simulink model "x3_2_F1_step_response"  (R2021b)
settings: Solver=VariableStepAuto  StartTime=0.0  StopTime=200  RelTol=1e-3
libraries: simulink x1
settings Model: Creator=Edwar  LastModifiedBy=Edwar

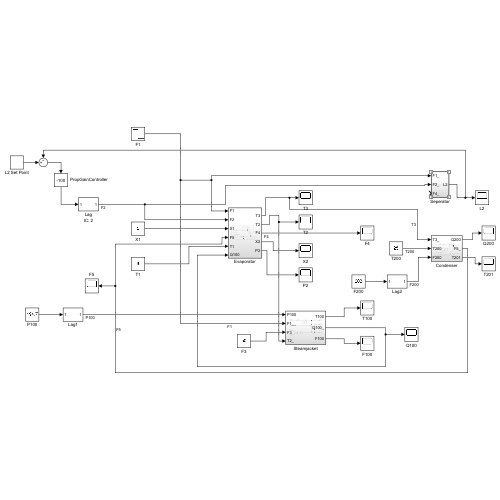
[thumbnail: Simulink's stored preview of the top-level diagram]
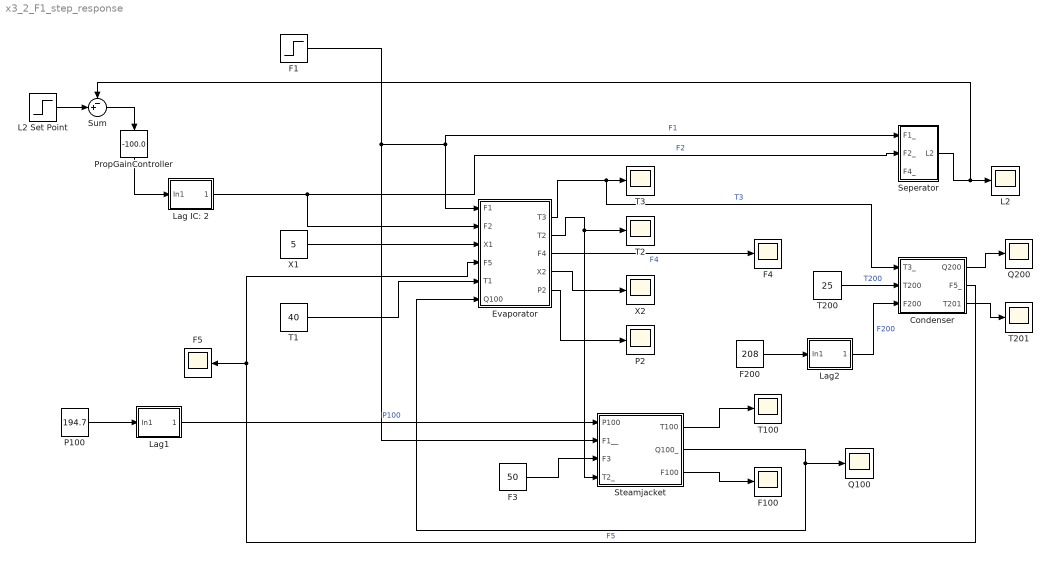
== system x3_2_F1_step_response ==
  Condenser : Subsystem
  Evaporator : Subsystem
  F1 : Step  Time=30  Before=10  After=9  SampleTime=0
  F100 : Scope
  F200 : Constant  Value=208
  F3 : Constant  Value=50
  F4 : Scope
  F5 : Scope
  L2 : Scope
  L2 Set Point : Step  Time=50  Before=1  SampleTime=0
  Lag IC: 2 : Subsystem
  Lag1 : Subsystem
  Lag2 : Subsystem
  P100 : Constant  Value=194.7
  P2 : Scope
  PropGainController : simulink/Math Operations/Slider Gain  gain=-100.0  low=-100  high=0
  Q100 : Scope
  Q200 : Scope
  Seperator : Subsystem
  Steamjacket : Subsystem
  Sum : Sum  Inputs=-+|
  T1 : Constant  Value=40
  T{2..3,100,201} (4 alike) : Scope
  T200 : Constant  Value=25
  X1 : Constant  Value=5
  X2 : Scope
  wires:
  Evaporator/2(T2) -> T2/1, Steamjacket/4(T2_)
  Steamjacket/3(F100) -> F100/1
  X1/1 -> Evaporator/3(X1)
  Evaporator/4(X2) -> X2/1
  F3/1 -> Steamjacket/3(F3)
  Steamjacket/2(Q100_) -> Q100/1, Evaporator/6(Q100)
  T1/1 -> Evaporator/5(T1)
  Condenser/1(Q200) -> Q200/1
  Evaporator/3(F4) -> F4/1  "F4"
  Evaporator/5(P2) -> P2/1
  T200/1 -> Condenser/2(T200)  "T200"
  Steamjacket/1(T100) -> T100/1
  Evaporator/1(T3) -> T3/1, Condenser/1(T3_)  "T3"
  Condenser/3(T201) -> T201/1
  F1/1 -> Steamjacket/2(F1__), Seperator/1(F1_), Evaporator/1(F1)  "F1"
  Condenser/2(F5_) -> Evaporator/4(F5), F5/1  "F5"
  Seperator/1(L2) -> Sum/1, L2/1
  Lag IC: 2/1(Output) -> Seperator/2(F2_), Evaporator/2(F2)  "F2"
  Lag1/1(Output) -> Steamjacket/1(P100)  "P100"
  P100/1 -> Lag1/1(In1)
  F200/1 -> Lag2/1(In1)
  Lag2/1(Output) -> Condenser/3(F200)  "F200"
  L2 Set Point/1 -> Sum/2
  Sum/1 -> PropGainController/1
  PropGainController/1 -> Lag IC: 2/1(In1)

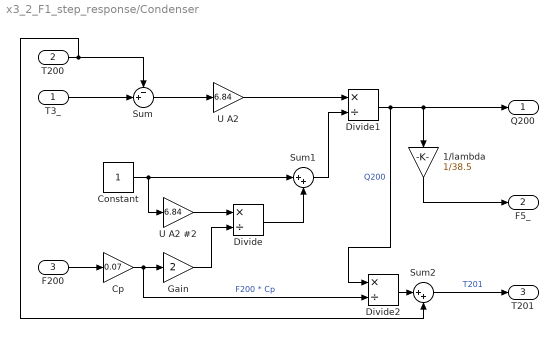
== system x3_2_F1_step_response/Condenser ==
  T3_ : Inport
  T200 : Inport  Port=2
  F200 : Inport  Port=3
  1/lambda : Gain  Gain=1/38.5
  Constant : Constant
  Cp : Gain  Gain=0.07
  Divide : Product  Inputs=*/
  Divide1 : Product  Inputs=*/
  Divide2 : Product  Inputs=*/
  Gain : Gain  Gain=2
  Sum : Sum  Inputs=-+|
  Sum1 : Sum  Inputs=|++
  Sum2 : Sum  Inputs=|++
  U A2 : Gain  Gain=6.84
  U A2 #2 : Gain  Gain=6.84
  Q200 : Outport
  F5_ : Outport  Port=2
  T201 : Outport  Port=3
  wires:
  Sum1/1 -> Divide1/2
  Gain/1 -> Divide/2
  T200/1 -> Sum2/2, Sum/1
  Divide/1 -> Sum1/2
  Divide1/1 -> Divide2/1, Q200/1, 1/lambda/1  "Q200"
  U A2/1 -> Divide1/1
  F200/1 -> Cp/1
  Sum/1 -> U A2/1
  Constant/1 -> U A2 #2/1, Sum1/1
  T3_/1 -> Sum/2
  U A2 #2/1 -> Divide/1
  Cp/1 -> Divide2/2, Gain/1  "F200 * Cp"
  1/lambda/1 -> F5_/1
  Sum2/1 -> T201/1  "T201"
  Divide2/1 -> Sum2/1

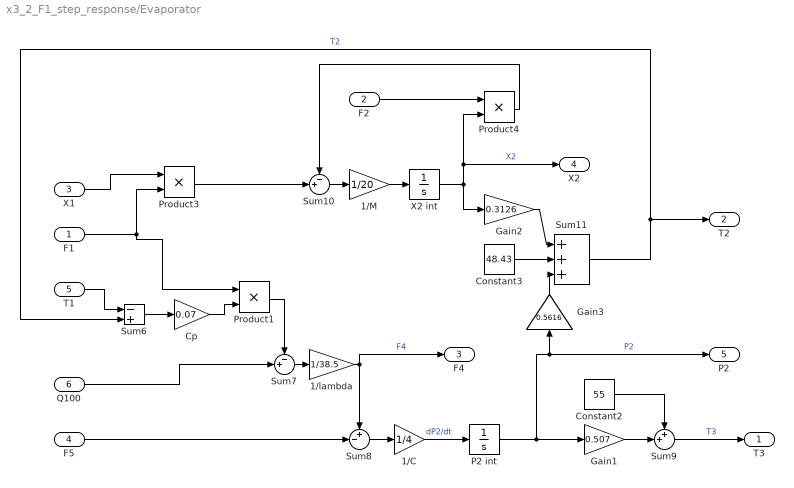
== system x3_2_F1_step_response/Evaporator ==
  F1 : Inport
  F2 : Inport  Port=2
  X1 : Inport  Port=3
  F5 : Inport  Port=4
  T1 : Inport  Port=5
  Q100 : Inport  Port=6
  1/C : Gain  Gain=1/4
  1/M : Gain  Gain=1/20
  1/lambda : Gain  Gain=1/38.5
  Constant2 : Constant  Value=55
  Constant3 : Constant  Value=48.43
  Cp : Gain  Gain=0.07
  Gain1 : Gain  Gain=0.507
  Gain2 : Gain  Gain=0.3126
  Gain3 : Gain  Gain=0.5616
  P2 int : Integrator
  Product1 : Product
  Product3 : Product
  Product4 : Product
  Sum10 : Sum  Inputs=-+|
  Sum11 : Sum  Inputs=+++
  Sum6 : Sum  Inputs=-+
  Sum7 : Sum  Inputs=-+|
  Sum8 : Sum  Inputs=+-|
  Sum9 : Sum  Inputs=++|
  X2 int : Integrator
  T3 : Outport
  T2 : Outport  Port=2
  F4 : Outport  Port=3
  X2 : Outport  Port=4
  P2 : Outport  Port=5
  wires:
  F2/1 -> Product4/1
  1/C/1 -> P2 int/1  "dP2/dt"
  Sum9/1 -> T3/1  "T3"
  1/M/1 -> X2 int/1
  Gain3/1 -> Sum11/3
  Constant3/1 -> Sum11/2
  Gain2/1 -> Sum11/1
  Constant2/1 -> Sum9/1
  Q100/1 -> Sum7/2
  X2 int/1 -> X2/1, Product4/2, Gain2/1  "X2"
  1/lambda/1 -> F4/1, Sum8/1  "F4"
  Sum11/1 -> T2/1, Sum6/2  "T2"
  Sum7/1 -> 1/lambda/1
  Product3/1 -> Sum10/2
  Product1/1 -> Sum7/1
  F1/1 -> Product1/1, Product3/2
  Gain1/1 -> Sum9/2
  Sum6/1 -> Cp/1
  Sum8/1 -> 1/C/1
  P2 int/1 -> P2/1, Gain3/1, Gain1/1  "P2"
  Sum10/1 -> 1/M/1
  Product4/1 -> Sum10/1
  Cp/1 -> Product1/2
  T1/1 -> Sum6/1
  X1/1 -> Product3/1
  F5/1 -> Sum8/2

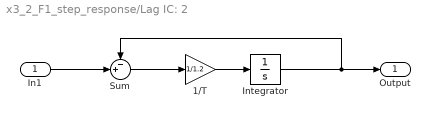
== system x3_2_F1_step_response/Lag IC: 2 ==
  In1 : Inport
  1/T : Gain  Gain=1/1.2
  Integrator : Integrator  InitialCondition=1
  Sum : Sum  Inputs=-+|
  Output : Outport
  wires:
  Integrator/1 -> Sum/1, Output/1
  Sum/1 -> 1/T/1
  1/T/1 -> Integrator/1
  In1/1 -> Sum/2

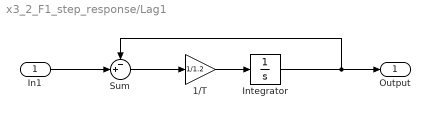
== system x3_2_F1_step_response/Lag1 ==
  In1 : Inport
  1/T : Gain  Gain=1/1.2
  Integrator : Integrator  InitialCondition=194.7
  Sum : Sum  Inputs=-+|
  Output : Outport
  wires:
  In1/1 -> Sum/2
  1/T/1 -> Integrator/1
  Sum/1 -> 1/T/1
  Integrator/1 -> Output/1, Sum/1

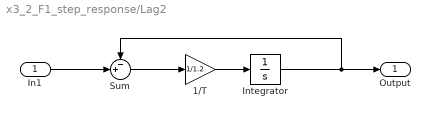
== system x3_2_F1_step_response/Lag2 ==
  In1 : Inport
  1/T : Gain  Gain=1/1.2
  Integrator : Integrator  InitialCondition=208
  Sum : Sum  Inputs=-+|
  Output : Outport
  wires:
  Integrator/1 -> Sum/1, Output/1
  Sum/1 -> 1/T/1
  1/T/1 -> Integrator/1
  In1/1 -> Sum/2

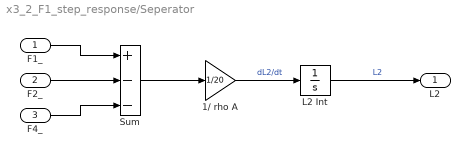
== system x3_2_F1_step_response/Seperator ==
  F1_ : Inport
  F2_ : Inport  Port=2
  F4_ : Inport  Port=3
  1/ rho A : Gain  Gain=1/20
  L2 Int : Integrator  InitialCondition=1
  Sum : Sum  Inputs=+--
  L2 : Outport
  wires:
  Sum/1 -> 1/ rho A/1
  L2 Int/1 -> L2/1  "L2"
  F4_/1 -> Sum/3
  F2_/1 -> Sum/2
  1/ rho A/1 -> L2 Int/1  "dL2/dt"
  F1_/1 -> Sum/1

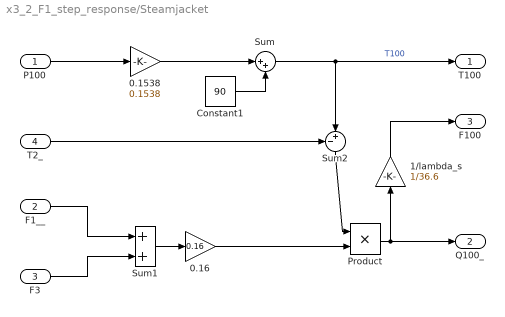
== system x3_2_F1_step_response/Steamjacket ==
  P100 : Inport
  F1__ : Inport  Port=2
  F3 : Inport  Port=3
  T2_ : Inport  Port=4
  0.1538 : Gain  Gain=0.1538
  0.16 : Gain  Gain=0.16
  1/lambda_s : Gain  Gain=1/36.6
  Constant1 : Constant  Value=90
  Product : Product
  Sum : Sum  Inputs=|++
  Sum1 : Sum
  Sum2 : Sum  Inputs=-+|
  T100 : Outport
  Q100_ : Outport  Port=2
  F100 : Outport  Port=3
  wires:
  Constant1/1 -> Sum/2
  1/lambda_s/1 -> F100/1
  T2_/1 -> Sum2/1
  Product/1 -> Q100_/1, 1/lambda_s/1
  0.1538/1 -> Sum/1
  Sum2/1 -> Product/1
  Sum/1 -> T100/1, Sum2/2  "T100"
  F1__/1 -> Sum1/1
  P100/1 -> 0.1538/1
  Sum1/1 -> 0.16/1
  0.16/1 -> Product/2
  F3/1 -> Sum1/2
